simulink model "exp3"  (R2023a)
settings: Solver=ode4  StartTime=0.0  StopTime=7  FixedStep=0.0001  RelTol=1e-3
values from neighbouring files (symbols this model uses):
  Bm = Br + B1/N^2    (= 0.00041)    [Example4_2.m]    (also in Example5_6_7_8.m = 0.000432222222222)
  Dis_Tq = 1    [Example5_6_7_8.m]
  g = 9.8    [Example5_6_7_8.m]
  Im = Ir + I1/N^2    (= 1.19e-05)    [Example4_2.m]    (also in Example5_6_7_8.m = 1.74555555556e-05)
  Ka = 8.22e-2    (= 0.0822)    [Example4_2.m]    (also in Example5_6_7_8.m)
  Ke = 8.24e-2    (= 0.0824)    [Example4_2.m]    (also in Example5_6_7_8.m)
  Kp = Omega_n/(2*Zeta)    [Example5_6_7_8.m]
  Kt = Ka*Kg    (= 0.0822)    [Example5_6_7_8.m]
  Ku = 1    [Example4_2.m]    (also in Example5_6_7_8.m = 3)
  Kv = 2*Zeta*Omega_n/Km    [Example5_6_7_8.m]
  L = 0.1    [Example5_6_7_8.m]
  La = 6.1e-4    (= 0.00061)    [Example4_2.m]    (also in Example5_6_7_8.m)
  m = 0.5    [Example5_6_7_8.m]
  N = 50    [Example4_2.m]    (also in Example5_6_7_8.m = 30)
  Ra = 2.49    [Example4_2.m]    (also in Example5_6_7_8.m)
  Tv = Tm    (= 0.038552377892)    [Example5_6_7_8.m]
settings Model: Creator=wyw  LastModifiedBy=wyw

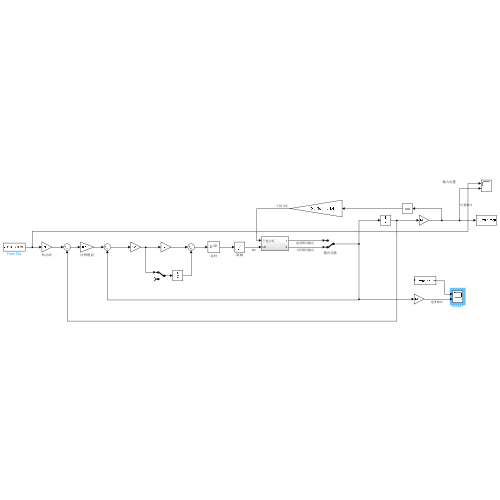
[thumbnail: Simulink's stored preview of the top-level diagram]
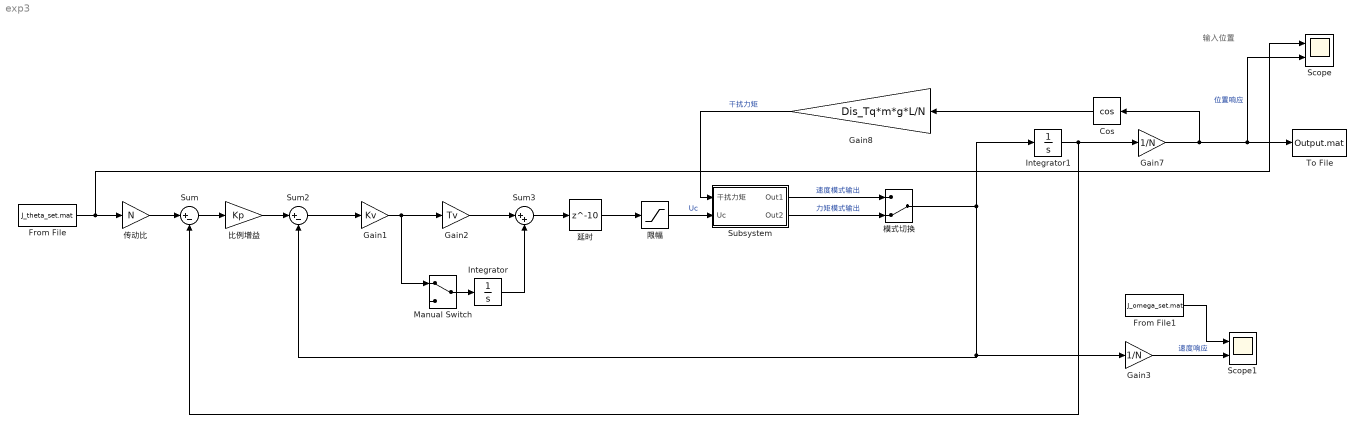
== system exp3 ==
  note: 输入位置
  Cos : Trigonometry  Operator=cos
  From File : FromFile  FileName=J_theta_set.mat  SampleTime=0
  From File1 : FromFile  FileName=J_omega_set.mat  SampleTime=0
  Gain1 : Gain  Gain=Kv
  Gain2 : Gain  Gain=Tv
  Gain3 : Gain  Gain=1/N
  Gain7 : Gain  Gain=1/N
  Gain8 : Gain  Gain=Dis_Tq*m*g*L/N
  Integrator : Integrator
  Integrator1 : Integrator
  Manual Switch : ManualSwitch
  Scope : Scope  NumInputPorts=2
  Scope1 : Scope  NumInputPorts=2
  Subsystem : Subsystem
  Sum : Sum  Inputs=|+-
  Sum2 : Sum  Inputs=|+-
  Sum3 : Sum  Inputs=|++
  To File : ToFile  Filename=Output.mat  SaveFormat=Timeseries
  传动比 : Gain  Gain=N
  延时 : Delay  DelayLength=10  InitialCondition=0
  模式切换 : ManualSwitch  CurrentSetting=0
  比例增益 : Gain  Gain=Kp
  限幅 : Saturate  UpperLimit=10  LowerLimit=-10
  wires:
  比例增益/1 -> Sum2/1
  传动比/1 -> Sum/1
  Sum/1 -> 比例增益/1
  Sum2/1 -> Gain1/1
  Manual Switch/1 -> Integrator/1
  Gain1/1 -> Manual Switch/1, Gain2/1
  Integrator/1 -> Sum3/2
  Gain2/1 -> Sum3/1
  Sum3/1 -> 延时/1
  延时/1 -> 限幅/1
  Integrator1/1 -> Sum/2, Gain7/1
  Gain7/1 -> Scope/2, To File/1, Cos/1  "位置响应"
  From File/1 -> Scope/1, 传动比/1
  Cos/1 -> Gain8/1
  模式切换/1 -> Integrator1/1, Sum2/2, Gain3/1
  Gain8/1 -> Subsystem/1(干扰力矩)  "干扰力矩"
  限幅/1 -> Subsystem/2(Uc)  "Uc"
  Subsystem/1(Out1) -> 模式切换/1  "速度模式输出"
  Subsystem/2(Out2) -> 模式切换/2  "力矩模式输出"
  From File1/1 -> Scope1/1
  Gain3/1 -> Scope1/2  "速度响应"

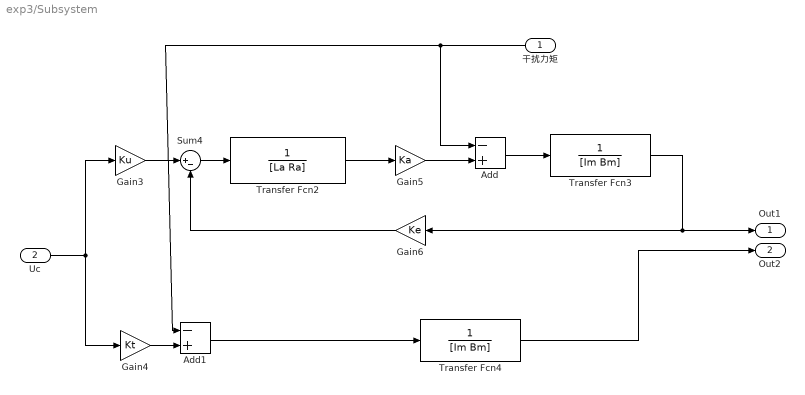
== system exp3/Subsystem ==
  干扰力矩 : Inport
  Uc : Inport  Port=2
  Add : Sum  Inputs=-+
  Add1 : Sum  Inputs=-+
  Gain3 : Gain  Gain=Ku
  Gain4 : Gain  Gain=Kt
  Gain5 : Gain  Gain=Ka
  Gain6 : Gain  Gain=Ke
  Sum4 : Sum  Inputs=|+-
  Transfer Fcn2 : TransferFcn  Denominator=[La Ra]
  Transfer Fcn3 : TransferFcn  Denominator=[Im Bm]
  Transfer Fcn4 : TransferFcn  Denominator=[Im Bm]
  Out1 : Outport
  Out2 : Outport  Port=2
  wires:
  Transfer Fcn2/1 -> Gain5/1
  干扰力矩/1 -> Add1/1, Add/1
  Gain3/1 -> Sum4/1
  Gain4/1 -> Add1/2
  Transfer Fcn3/1 -> Out1/1, Gain6/1
  Add1/1 -> Transfer Fcn4/1
  Uc/1 -> Gain4/1, Gain3/1
  Add/1 -> Transfer Fcn3/1
  Sum4/1 -> Transfer Fcn2/1
  Gain5/1 -> Add/2
  Gain6/1 -> Sum4/2
  Transfer Fcn4/1 -> Out2/1
